simulink model "integrate_psd"  (Simulink 6.3)
settings: Solver=ode3  StartTime=0.0  StopTime=ww(end)  FixedStep=min(diff(ww))  RelTol=1e-3
settings Model: LastModifiedBy=E704491

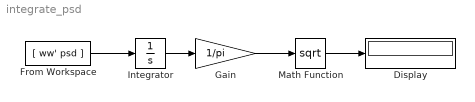
== system integrate_psd ==
  Display : Display
  From Workspace : FromWorkspace  VariableName=[ ww' psd ]  SampleTime=0
  Gain : Gain  Gain=1/pi
  Integrator : Integrator
  Math Function : Math  Operator=sqrt  SaturateOnIntegerOverflow=on
  wires:
  From Workspace/1 -> Integrator/1
  Integrator/1 -> Gain/1
  Gain/1 -> Math Function/1
  Math Function/1 -> Display/1
